simulink model "mpc_no_load_R2020a"  (R2020a)
settings: Solver=ode3  StartTime=0.0  StopTime=inf  FixedStep=Ts_sim  RelTol=1e-3
InitFcn:
  | ros_init_callback
values from neighbouring files (symbols this model uses):
  max_vel_xy = 5    [initialise_iris_gains.m]
  max_vel_z_down = 5    [initialise_iris_gains.m]
  max_vel_z_up = 5    [initialise_iris_gains.m]
  MPC_ACC_DOWN_MAX = 3    [initialise_iris_gains.m]
  MPC_ACC_HOR_MAX = 5    [initialise_iris_gains.m]
  MPC_ACC_UP_MAX = 4    [initialise_iris_gains.m]
  MPC_XY_VEL_D_ACC = 0.2    [initialise_iris_gains.m]
  MPC_XY_VEL_I_ACC = 0.4    [initialise_iris_gains.m]
  MPC_XY_VEL_P_ACC = 1.8    [initialise_iris_gains.m]
  MPC_Z_VEL_D_ACC = 0    [initialise_iris_gains.m]
  MPC_Z_VEL_I_ACC = 2    [initialise_iris_gains.m]
  MPC_Z_VEL_P_ACC = 4    [initialise_iris_gains.m]
  Ts_pos_control = 0.01    [initialise_ros_iris_payload.m]    (also in ros_init_callback.m)
undefined symbols (not defined in the file or in its folder): DiscIntNeverNeededParam, q_int_lim, u_bar, vel_filt_denom, vel_filt_num, X, Y, Z
libraries: robotlib x3, simulink x3, robotgazebolib x1, mpclib x1
settings Model: Creator=esl  LastModifiedBy=murray
settings OptimizationCC: EnhancedBackFolding=on  PassReuseOutputArgsAs=Individual arguments  ZeroExternalMemoryAtStartup=off  ZeroInternalMemoryAtStartup=off  MaxStackSize=64  OptimizeBlockOrder=speed  DifferentSizesBufferReuse=on  OptimizationCustomize=off  EfficientTunableParamExpr=on
settings DebuggingCC: ParameterTunabilityLossMsg=error  SFMachineParentedDataDiag=error
settings HardwareCC: ProdBitPerLong=64  ProdHWDeviceType=Intel->x86-64 (Linux 64)  UseEmbeddedCoderFeatures=off
settings SFSimCC: MATLABDynamicMemAlloc=off
settings RTWCC: SystemTargetFile=ert.tlc  HardwareBoard=Robot Operating System (ROS)  TemplateMakefile=ert_default_tmf  Toolchain=Catkin  TargetLang=C++
settings CodeAppCC: ForceParamTrailComments=on  IgnoreCustomStorageClasses=off  OperatorAnnotations=on  SimulinkDataObjDesc=on  SFDataObjDesc=on  InsertBlockDesc=on
settings ERTTargetCC: SupportNonInlinedSFcns=on

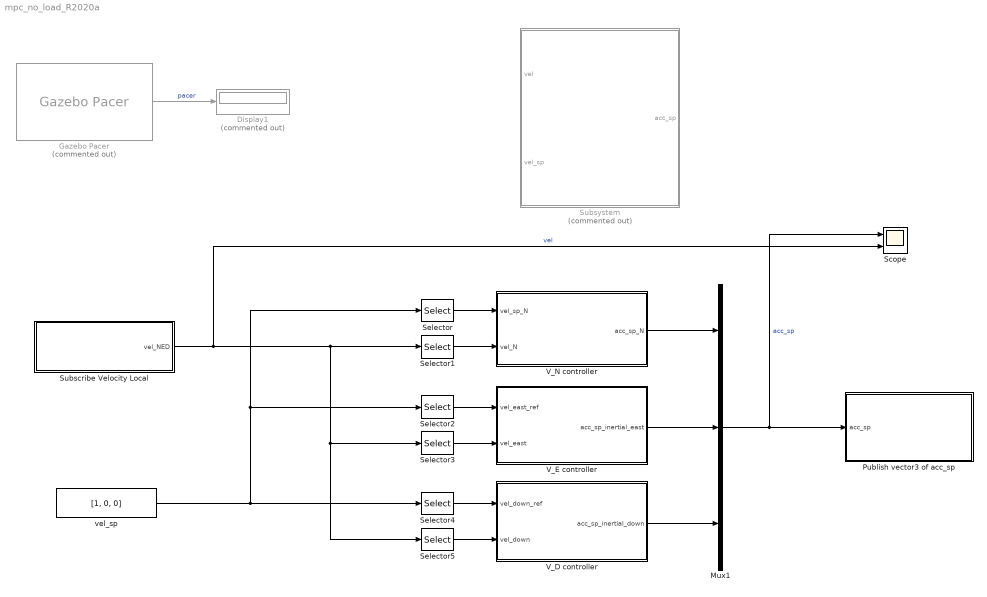
== system mpc_no_load_R2020a ==
  Display1 : Display  Commented=on
  Gazebo Pacer : robotgazebolib/Gazebo Pacer  Commented=on  ResetBehavior=Reset Gazebo simulation time  SampleTime=0.004
      settings: SourceProductBaseCode=RO
  Mux1 : Mux  Inputs=3
  Publish vector3 of acc_sp : Subsystem
  Scope : Scope  NumInputPorts=2
  Selector : Selector  InputPortWidth=3  IndexOptions=Index vector (dialog)  Indices=1  OutputSizes=1
  Selector1 : Selector  InputPortWidth=3  IndexOptions=Index vector (dialog)  Indices=1  OutputSizes=1
  Selector2 : Selector  InputPortWidth=3  IndexOptions=Index vector (dialog)  Indices=2  OutputSizes=1
  Selector3 : Selector  InputPortWidth=3  IndexOptions=Index vector (dialog)  Indices=2  OutputSizes=1
  Selector4 : Selector  InputPortWidth=3  IndexOptions=Index vector (dialog)  Indices=3  OutputSizes=1
  Selector5 : Selector  InputPortWidth=3  IndexOptions=Index vector (dialog)  Indices=3  OutputSizes=1
  Subscribe Velocity Local : Subsystem
  Subsystem : Subsystem  Commented=on
  V_D controller : Subsystem
  V_E controller : Subsystem
  V_N controller : Subsystem
  vel_sp : Constant  Value=[1, 0, 0]
  wires:
  Gazebo Pacer/1 -> Display1/1  "pacer"
  V_D controller/1(acc_sp_inertial_down) -> Mux1/3
  V_E controller/1(acc_sp_inertial_east) -> Mux1/2
  V_N controller/1(acc_sp_N) -> Mux1/1
  Selector/1 -> V_N controller/1(vel_sp_N)
  Selector1/1 -> V_N controller/2(vel_N)
  Selector5/1 -> V_D controller/2(vel_down)
  Selector4/1 -> V_D controller/1(vel_down_ref)
  Selector3/1 -> V_E controller/2(vel_east)
  Selector2/1 -> V_E controller/1(vel_east_ref)
  Subscribe Velocity Local/1(vel_NED) -> Scope/2, Selector3/1, Selector5/1, Selector1/1  "vel"
  vel_sp/1 -> Selector2/1, Selector/1, Selector4/1
  Mux1/1 -> Publish vector3 of acc_sp/1(acc_sp), Scope/1  "acc_sp"

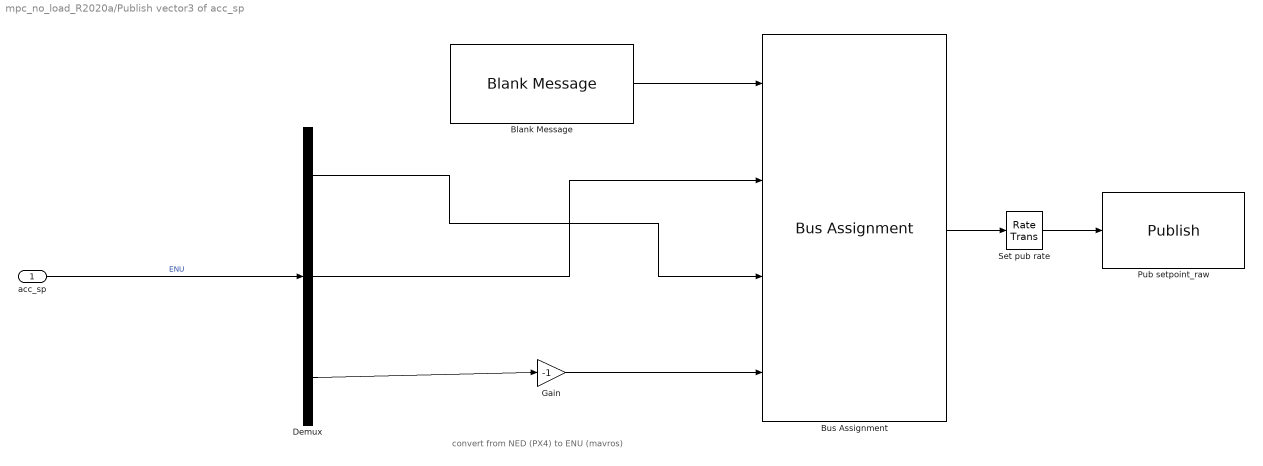
== system mpc_no_load_R2020a/Publish vector3 of acc_sp ==
  note: convert from NED (PX4) to ENU (mavros)
  acc_sp : Inport
  Blank Message : robotlib/Blank Message  messageClass=Message  entityType=geometry_msgs/Vector3  messageType=geometry_msgs/Vector3  SampleTime=inf
  Bus Assignment : BusAssignment  AssignedSignals=X,Y,Z
  Demux : Demux  Outputs=3
  Gain : Gain  Gain=-1
  Pub setpoint_raw : robotlib/Publish  topicSource=Specify your own  topic=/simulink/acc_sp  messageType=geometry_msgs/Vector3  messageQueueLength=1
  Set pub rate : RateTransition  OutPortSampleTime=Ts_publish
  wires:
  Set pub rate/1 -> Pub setpoint_raw/1
  Bus Assignment/1 -> Set pub rate/1
  Blank Message/1 -> Bus Assignment/1
  Demux/1 -> Bus Assignment/3
  Demux/2 -> Bus Assignment/2
  Demux/3 -> Gain/1
  Gain/1 -> Bus Assignment/4
  acc_sp/1 -> Demux/1  "ENU"

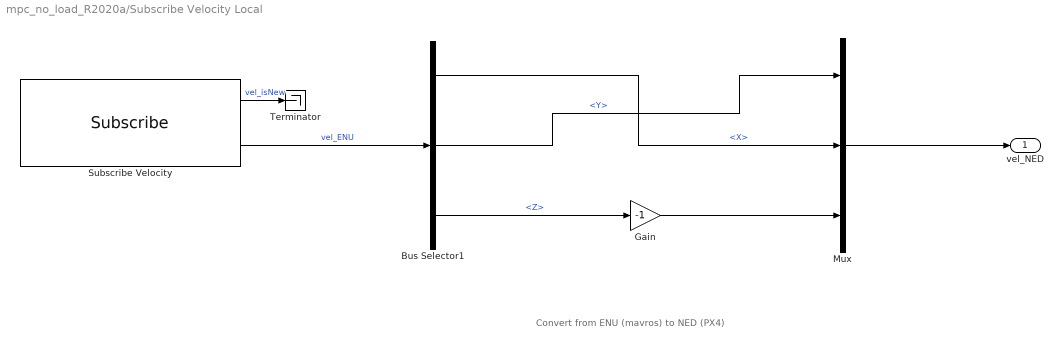
== system mpc_no_load_R2020a/Subscribe Velocity Local ==
  note: Convert from ENU (mavros) to NED (PX4)
  Bus Selector1 : BusSelector  OutputSignals=Twist.Linear.X,Twist.Linear.Y,Twist.Linear.Z
  Gain : Gain  Gain=-1
  Mux : Mux  Inputs=3
  Subscribe Velocity : robotlib/Subscribe  topicSource=Select from ROS network  topic=/mavros/local_position/velocity_local  messageType=geometry_msgs/TwistStamped  sampleTime=Ts_sub  messageQueueLength=1
  Terminator : Terminator
  vel_NED : Outport
  wires:
  Subscribe Velocity/1 -> Terminator/1  "vel_isNew"
  Subscribe Velocity/2 -> Bus Selector1/1  "vel_ENU"
  Mux/1 -> vel_NED/1
  Bus Selector1/1 -> Mux/2  "<X>"
  Bus Selector1/2 -> Mux/1  "<Y>"
  Bus Selector1/3 -> Gain/1  "<Z>"
  Gain/1 -> Mux/3

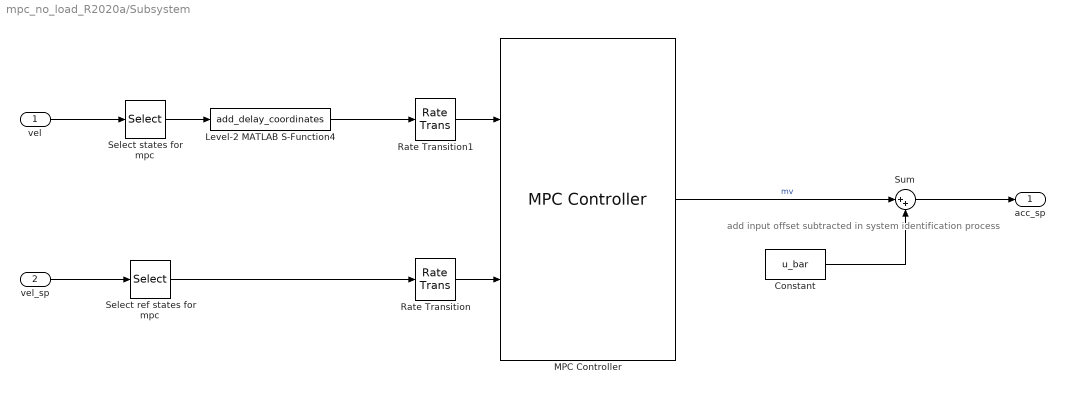
== system mpc_no_load_R2020a/Subsystem ==
  note: add input offset subtracted in system identification process
  vel : Inport
  vel_sp : Inport  Port=2
  Constant : Constant  Value=u_bar
  Level-2 MATLAB S-Function4 : M-S-Function  FunctionName=add_delay_coordinates  Parameters=y_ext_0, q, Ts_mpc, ny
  MPC Controller : mpclib/MPC Controller  SCDEnableBlockLinearizationSpecification=on  mpcobj=mpc_vel  is_multiple=0  enable_value=0  return_u0=off  updateMPCinCallerWorkspace=on  md_inport=off  mv_inport=off  uref_inport=off  return_cost=off  return_mvseq=off  return_qpstatus=off  return_xseq=off  return_state=off  return_ovseq=off  state_inport=off  umin_inport=off  umax_inport=off  ymin_inport=off  ymax_inport=off  cc_inport=off  ywt_inport=off  uwt_inport=off  duwt_inport=off  rhoeps_inport=off  pm_inport=off  MaximumP=10  HorizonChoice=FixedHorizon  n_ts=0.03  n_p=266  n_mv=1  n_md=0  n_ud=0  n_mo=42  n_uo=1  BlockDataType=double  SampleTimeInherited=off  switch_inport=off
  Rate Transition : RateTransition  Deterministic=off  OutPortSampleTime=Ts_mpc
  Rate Transition1 : RateTransition  Deterministic=off  OutPortSampleTime=Ts_mpc
  Select ref states for mpc : Selector  InputPortWidth=3  IndexOptions=Index vector (dialog)  Indices=mpc_states  OutputSizes=1
  Select states for mpc : Selector  InputPortWidth=3  IndexOptions=Index vector (dialog)  Indices=mpc_states  OutputSizes=1
  Sum : Sum  Inputs=|++
  acc_sp : Outport  OutDataTypeStr=double  PortDimensions=nu
  wires:
  vel/1 -> Select states for mpc/1
  vel_sp/1 -> Select ref states for mpc/1
  Sum/1 -> acc_sp/1
  Select states for mpc/1 -> Level-2 MATLAB S-Function4/1
  MPC Controller/1 -> Sum/1  "mv"
  Level-2 MATLAB S-Function4/1 -> Rate Transition1/1
  Select ref states for mpc/1 -> Rate Transition/1
  Constant/1 -> Sum/2
  Rate Transition1/1 -> MPC Controller/1
  Rate Transition/1 -> MPC Controller/2

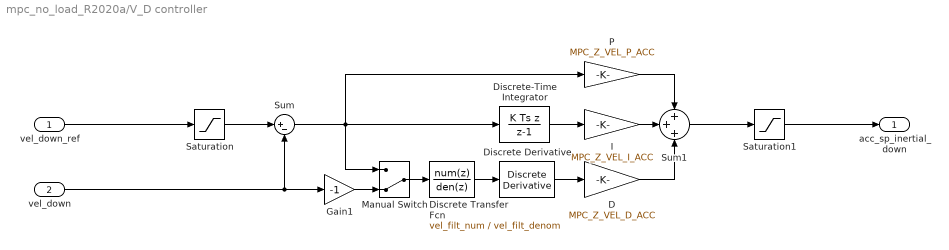
== system mpc_no_load_R2020a/V_D controller ==
  vel_down_ref : Inport  SampleTime=Ts_pos_control
  vel_down : Inport  Port=2  SampleTime=Ts_pos_control
  D : Gain  Gain=MPC_Z_VEL_D_ACC
  Discrete Transfer Fcn : DiscreteTransferFcn  Numerator=vel_filt_num  Denominator=vel_filt_denom
  Discrete Derivative : simulink/Discrete/Discrete Derivative  gainval=1  ICPrevScaledInput=0.0  OutMin=[]  OutMax=[]  OutDataType=fixdt(1, 16)  OutScaling=2^-10  DoSatur=off
  Discrete-Time Integrator : DiscreteIntegrator  IntegratorMethod=Integration: Backward Euler  gainval=1  SampleTime=-1  UpperSaturationLimit=q_int_lim  LowerSaturationLimit=-q_int_lim  ICPrevOutput=DiscIntNeverNeededParam  ICPrevScaledInput=DiscIntNeverNeededParam
  Gain1 : Gain  Gain=-1
  I : Gain  Gain=MPC_Z_VEL_I_ACC
  Manual Switch : ManualSwitch  CurrentSetting=0
  P : Gain  Gain=MPC_Z_VEL_P_ACC
  Saturation : Saturate  UpperLimit=max_vel_z_up  LowerLimit=-abs(max_vel_z_down)
  Saturation1 : Saturate  UpperLimit=MPC_ACC_UP_MAX  LowerLimit=-MPC_ACC_DOWN_MAX
  Sum : Sum  Inputs=|+-
  Sum1 : Sum  Inputs=+++
  acc_sp_inertial_down : Outport  VectorParamsAs1DForOutWhenUnconnected=off
  wires:
  vel_down_ref/1 -> Saturation/1
  Discrete Derivative/1 -> D/1
  I/1 -> Sum1/2
  D/1 -> Sum1/3
  vel_down/1 -> Gain1/1, Sum/2
  P/1 -> Sum1/1
  Sum/1 -> Discrete-Time Integrator/1, Manual Switch/1, P/1
  Discrete Transfer Fcn/1 -> Discrete Derivative/1
  Gain1/1 -> Manual Switch/2
  Saturation/1 -> Sum/1
  Discrete-Time Integrator/1 -> I/1
  Sum1/1 -> Saturation1/1
  Manual Switch/1 -> Discrete Transfer Fcn/1
  Saturation1/1 -> acc_sp_inertial_down/1

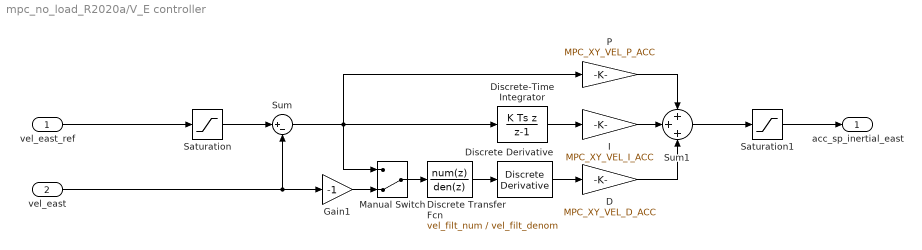
== system mpc_no_load_R2020a/V_E controller ==
  vel_east_ref : Inport  SampleTime=Ts_pos_control
  vel_east : Inport  Port=2  SampleTime=Ts_pos_control
  D : Gain  Gain=MPC_XY_VEL_D_ACC
  Discrete Transfer Fcn : DiscreteTransferFcn  Numerator=vel_filt_num  Denominator=vel_filt_denom
  Discrete Derivative : simulink/Discrete/Discrete Derivative  gainval=1  ICPrevScaledInput=0.0  OutMin=[]  OutMax=[]  OutDataType=fixdt(1, 16)  OutScaling=2^-10  DoSatur=off
  Discrete-Time Integrator : DiscreteIntegrator  IntegratorMethod=Integration: Backward Euler  gainval=1  SampleTime=-1  UpperSaturationLimit=q_int_lim  LowerSaturationLimit=-q_int_lim  ICPrevOutput=DiscIntNeverNeededParam  ICPrevScaledInput=DiscIntNeverNeededParam
  Gain1 : Gain  Gain=-1
  I : Gain  Gain=MPC_XY_VEL_I_ACC
  Manual Switch : ManualSwitch  CurrentSetting=0
  P : Gain  Gain=MPC_XY_VEL_P_ACC
  Saturation : Saturate  UpperLimit=max_vel_xy  LowerLimit=-max_vel_xy
  Saturation1 : Saturate  UpperLimit=MPC_ACC_HOR_MAX  LowerLimit=-MPC_ACC_HOR_MAX
  Sum : Sum  Inputs=|+-
  Sum1 : Sum  Inputs=+++
  acc_sp_inertial_east : Outport  VectorParamsAs1DForOutWhenUnconnected=off
  wires:
  vel_east/1 -> Gain1/1, Sum/2
  Discrete-Time Integrator/1 -> I/1
  Sum/1 -> Discrete-Time Integrator/1, Manual Switch/1, P/1
  vel_east_ref/1 -> Saturation/1
  Sum1/1 -> Saturation1/1
  Saturation/1 -> Sum/1
  Discrete Transfer Fcn/1 -> Discrete Derivative/1
  Discrete Derivative/1 -> D/1
  I/1 -> Sum1/2
  Manual Switch/1 -> Discrete Transfer Fcn/1
  Gain1/1 -> Manual Switch/2
  P/1 -> Sum1/1
  D/1 -> Sum1/3
  Saturation1/1 -> acc_sp_inertial_east/1

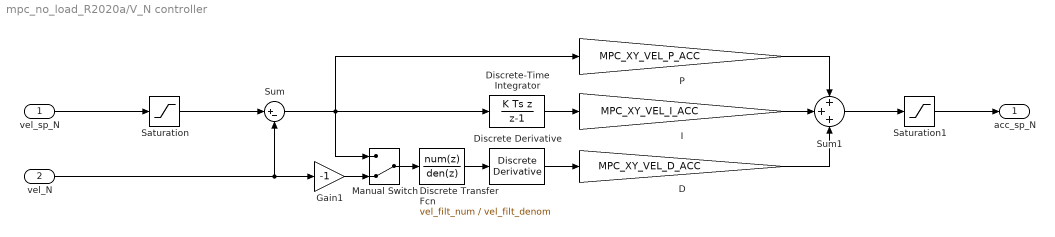
== system mpc_no_load_R2020a/V_N controller ==
  vel_sp_N : Inport  SampleTime=Ts_pos_control
  vel_N : Inport  Port=2  SampleTime=Ts_pos_control
  D : Gain  Gain=MPC_XY_VEL_D_ACC
  Discrete Transfer Fcn : DiscreteTransferFcn  Numerator=vel_filt_num  Denominator=vel_filt_denom
  Discrete Derivative : simulink/Discrete/Discrete Derivative  gainval=1  ICPrevScaledInput=0.0  OutMin=[]  OutMax=[]  OutDataType=fixdt(1, 16)  OutScaling=2^-10  DoSatur=off
  Discrete-Time Integrator : DiscreteIntegrator  IntegratorMethod=Integration: Backward Euler  gainval=1  SampleTime=-1  UpperSaturationLimit=max_vel_xy  LowerSaturationLimit=-max_vel_xy  ICPrevOutput=DiscIntNeverNeededParam  ICPrevScaledInput=DiscIntNeverNeededParam
  Gain1 : Gain  Gain=-1
  I : Gain  Gain=MPC_XY_VEL_I_ACC
  Manual Switch : ManualSwitch  CurrentSetting=0
  P : Gain  Gain=MPC_XY_VEL_P_ACC
  Saturation : Saturate  UpperLimit=max_vel_xy  LowerLimit=-max_vel_xy
  Saturation1 : Saturate  UpperLimit=MPC_ACC_HOR_MAX  LowerLimit=-MPC_ACC_HOR_MAX
  Sum : Sum  Inputs=|+-
  Sum1 : Sum  Inputs=+++
  acc_sp_N : Outport  VectorParamsAs1DForOutWhenUnconnected=off
  wires:
  vel_N/1 -> Gain1/1, Sum/2
  vel_sp_N/1 -> Saturation/1
  I/1 -> Sum1/2
  Sum/1 -> Manual Switch/1, Discrete-Time Integrator/1, P/1
  P/1 -> Sum1/1
  Sum1/1 -> Saturation1/1
  Discrete Derivative/1 -> D/1
  Discrete Transfer Fcn/1 -> Discrete Derivative/1
  D/1 -> Sum1/3
  Saturation/1 -> Sum/1
  Manual Switch/1 -> Discrete Transfer Fcn/1
  Discrete-Time Integrator/1 -> I/1
  Gain1/1 -> Manual Switch/2
  Saturation1/1 -> acc_sp_N/1
